simulink model "Ctrl_For_HRV_20260625_before_guidance_fix"  (R2024b)
settings: Solver=ode4  StartTime=0.0  StopTime=300  FixedStep=0.02  RelTol=1e-3
InitFcn:
  | Parameter;
values from neighbouring files (symbols this model uses):
  h_alpha = h_1    (= 0.02)    [Parameter.m]
  h_beta = h_1    (= 0.02)    [Parameter.m]
  h_miu = h_1    (= 0.02)    [Parameter.m]
  h_p = h_1    (= 0.02)    [Parameter.m]
  h_q = h_1    (= 0.02)    [Parameter.m]
  h_r = h_1    (= 0.02)    [Parameter.m]
  r_alpha = r_1    (= 0.04)    [Parameter.m]
  r_beta = r_1    (= 0.04)    [Parameter.m]
  r_miu = r_3    (= 0.03)    [Parameter.m]
  r_p = r_2    (= 1.28)    [Parameter.m]
  r_q = r_2    (= 1.28)    [Parameter.m]
  r_r = r_2    (= 1.28)    [Parameter.m]
  xishu = 0    [Parameter.m]
  xishu_D_0 = 0.3    [Parameter.m]
  xishu_L_0 = 0.2    [Parameter.m]
  xishu_l_0 = 0.23    [Parameter.m]
  xishu_m_0 = 0.17    [Parameter.m]
  xishu_n_0 = 0.09    [Parameter.m]
  xishu_Y_0 = 0.14    [Parameter.m]
undefined symbols (not defined in the file or in its folder): CCI_DUI_AngleRate_Controller, CCI_DUI_FlowAngle_Controller, fhan, PNG_2026_6_23
libraries: simulink x12
(part 2 of 2)

== matlab function Ctrl_For_HRV_20260625_before_guidance_fix/PNG/MATLAB Function1 ==
  data: ny_cmd input; alpha_cmd output; nz_cmd input; miu_cmd output; Q input; H input; Ma input; miu_last input
function [alpha_cmd, miu_cmd] = fcn(ny_cmd,nz_cmd,Q, H, Ma, miu_last)
%%%%%%%%%该函数的作用为将过载指令转化为攻角指令与倾侧角指令
%%
%参数设置
S = 334.73;
m = 63504;
earth_r = 6371000;
g0 = 9.8060;
R = earth_r+H; %R为地心距
g = (earth_r/R)^2*g0;
%% ===== 倾侧角 =====
nL=sqrt(ny_cmd^2+nz_cmd^2);
if nL <1e-4
    miu_cmd = miu_last;
else
    % atan2(y, z)，对应：
    % ny_cmd = n_lift_cmd * sin(miu_cmd)
    % nz_cmd = n_lift_cmd * cos(miu_cmd)
    miu_raw = atan2(ny_cmd, nz_cmd)

    % ===== 倾侧角连续化处理，避免 +pi/-pi 跳变 =====
    d_miu = miu_raw - miu_last;
    d_miu = mod(d_miu + pi, 2*pi) - pi;

    miu_cmd = miu_last + d_miu;
end
miu_cmd = mod(miu_cmd + pi, 2*pi) - pi;
% miu_cmd = -miu_cmd;
% miu_cmd = atan2(-ny_cmd, nz_cmd);

% if abs(miu_cmd) > pi / 2
%     miu_cmd = atan2(sin(miu_cmd - sign(miu_cmd) * pi), ...
%                 cos(miu_cmd - sign(miu_cmd) * pi));
%     % nL = -nL;
% else
%     miu_cmd = miu_cmd;
%     % nL = nL;
% end
%% ===== 攻角 =====
% C_L_alpha = (-8.19e-2)+(4.7e-2)*Ma+(1.86e-2)*alpha_deg-(4.73e-4)*(alpha_deg*Ma)-(9.19e-3)*Ma^2-(1.52e-4)*alpha_deg^2+(5.99e-7)*(alpha_deg*Ma)^2+(7.74e-4)*Ma^3+(4.08e-6)*alpha_deg^3-(2.93e-5)*Ma^4+(4.12e-7)*Ma^5;
% C_L_delta_a = (-1.45e-5)+(1.01e-4)*alpha_deg+(7.10e-6)*Ma-(4.14e-4)*delta_a-(3.51e-6)*(alpha_deg*delta_a)+(4.70e-6)*(alpha_deg*Ma)+(8.72e-6)*(Ma*delta_a)-(1.70e-7)*(alpha_deg*Ma)*delta_a;
% C_L_delta_e = (-1.45e-5)+(1.01e-4)*alpha_deg+(7.10e-6)*Ma-(4.14e-4)*delta_e-(3.51e-6)*(alpha_deg*delta_e)+(4.70e-6)*(alpha_deg*Ma)+(8.72e-6)*(Ma*delta_e)-(1.70e-7)*(alpha_deg*Ma)*delta_e;

%单位是角度
alpha_min = -30;
alpha_max = 30;

% CL_func = @(alpha_deg) (-8.19e-2)+(4.7e-2)*Ma+(1.86e-2)*alpha_deg-(4.73e-4)*(alpha_deg*Ma)-(9.19e-3)*Ma^2-(1.52e-4)*alpha_deg^2+(5.99e-7)*(alpha_deg*Ma)^2+(7.74e-4)*Ma^3+(4.08e-6)*alpha_deg^3-(2.93e-5)*Ma^4+(4.12e-7)*Ma^5 + ...
%                         (-1.45e-5)+(1.01e-4)*alpha_deg+(7.10e-6)*Ma-(4.14e-4)*delta_a-(3.51e-6)*(alpha_deg*delta_a)+(4.70e-6)*(alpha_deg*Ma)+(8.72e-6)*(Ma*delta_a)-(1.70e-7)*(alpha_deg*Ma)*delta_a + ...
%                         (-1.45e-5)+(1.01e-4)*alpha_deg+(7.10e-6)*Ma-(4.14e-4)*delta_e-(3.51e-6)*(alpha_deg*delta_e)+(4.70e-6)*(alpha_deg*Ma)+(8.72e-6)*(Ma*delta_e)-(1.70e-7)*(alpha_deg*Ma)*delta_e;

CL_func = @(alpha_deg) (-8.19e-2)+(4.7e-2)*Ma+(1.86e-2)*alpha_deg-(4.73e-4)*(alpha_deg*Ma)-(9.19e-3)*Ma^2-(1.52e-4)*alpha_deg^2+(5.99e-7)*(alpha_deg*Ma)^2+(7.74e-4)*Ma^3+(4.08e-6)*alpha_deg^3-(2.93e-5)*Ma^4+(4.12e-7)*Ma^5;
CL_min = CL_func(alpha_min);
CL_max = CL_func(alpha_max);

% ===== 目标CL =====

CL_cmd = nL*m*g/(Q*S);

% ===== 限制CL（关键）=====
CL_cmd = min(max(CL_cmd, CL_min), CL_max);

% ===== 求解 =====
alpha_cmd = fzero(@(a) CL_func(a) - CL_cmd, [alpha_min, alpha_max]);

%%

== matlab function Ctrl_For_HRV_20260625_before_guidance_fix/PNG/MATLAB Function2 ==
  data: V input; f_psi output; theta input; psi input; lat input; H input
function f_psi = earth_rotation(V,theta,psi,lat,H)

earth_r = 6371000;
w_e = 7.292116000000000e-05;
R = earth_r + H;
f_psi = V*cos(theta)*sin(psi)*tan(lat)/R ...
      + 2*w_e*(sin(lat)-cos(lat)*cos(psi)*tan(theta)) ...
      + w_e^2*R*cos(lat)*sin(lat)*sin(psi)/(V*cos(theta));

== matlab function Ctrl_For_HRV_20260625_before_guidance_fix/MATLAB Function2 ==
  data: position_t input; ny output; vt input; hgv_states input; theta_f input; kai_f input; nz output
function [ny, nz] = Prop_guidance(position_t, vt, hgv_states, theta_f, kai_f)
%--------------------------------------------------------------------------
% 两个平面的比例导引
% X-Y-Z 为北-天-东坐标系
% kai 在 x 轴右侧为正
%
% 输入：
%   xt, yt, zt   : 目标位置
%   gammat       : 目标航迹倾角
%   kait         : 目标航向角
%   Vt           : 目标速度
%   hgv_states   : [R, lon, lat, V, gamma, kai, x, y, z]
%   theta_f      : 期望终端弹道倾角
%   kai_f        : 期望终端航向角
%
% 输出：
%   ny           : 纵向过载
%   nz           : 侧向过载
%   out          : 中间变量，便于调试
%--------------------------------------------------------------------------

    %-----------------------------
    % 1. 读取状态量
    %-----------------------------
    H     = hgv_states(1);
    lon   = hgv_states(2); %#ok<NASGU>
    lat   = hgv_states(3);
    V     = hgv_states(4);
    gamma = hgv_states(5);
    kai   = hgv_states(6);
    x     = hgv_states(7);
    y     = hgv_states(8);
    z     = hgv_states(9);
    
    xt = position_t(1);
    yt = position_t(3);
    zt = position_t(2);
    %-----------------------------
    % 2. 常数与重力
    %-----------------------------
    earth_r = 6371000;
    g0 = 9.806000000000000;
    R = earth_r+H; %R_to_earth为地心距
    g = (earth_r/R)^2*g0;

    OMEGA_EARTH = 7.292116e-5;
    omega = OMEGA_EARTH;

    %-----------------------------
    % 3. 相对位置
    %-----------------------------
    rx = xt - x;
    ry = yt - y;
    rz = zt - z;

    %-----------------------------
    % 4. 目标速度分量
    % 这里保持你的 Python 代码逻辑，虽然后面没有直接用到
    %-----------------------------
    % vxt = Vt * cos(gammat) * cos(kait); %#ok<NASGU>
    % vyt = Vt * sin(gammat);             %#ok<NASGU>
    % vzt = Vt * cos(gammat) * sin(kait); %#ok<NASGU>
    vxt = vt(1);
    vyt = vt(3);
    vzt = vt(2);

    %-----------------------------
    % 5. 飞行器速度分量
    % 这里保持你的 Python 代码逻辑，虽然后面没有直接用到
    %-----------------------------
    vx = V * cos(gamma) * cos(kai); %#ok<NASGU>
    vy = V * sin(gamma);            %#ok<NASGU>
    vz = V * cos(gamma) * sin(kai); %#ok<NASGU>

    %-----------------------------
    % 6. 距离与视线角
    %-----------------------------
    rd = sqrt(rx^2 + ry^2 + rz^2);
    rc = sqrt(rx^2 + rz^2);

    qz = atan2(rz, rx);

    % Python 里是 atan(ry / rc)
    % MATLAB 里建议写成 atan2(ry, rc)，数值上更稳
    qy = atan2(ry, rc);

    % 如果想和 Python 完全一致，也可以改成：
    % qy = atan(ry / rc);

    %-----------------------------
    % 7. 视线角速度与距离变化率
    %-----------------------------
    qy_dot = -V * ( ...
        sin(gamma) * cos(qy) ...
        - cos(gamma) * sin(qy) * cos(kai - qz) ...
        ) / rd;

    qz_dot = -V * cos(gamma) * sin(kai - qz) / ...
        (rd * cos(qy));

    rd_dot = -V * ( ...
        cos(gamma) * cos(qy) * cos(kai - qz) ...
        + sin(gamma) * sin(qy) ...
        );

    %-----------------------------
    % 8. 剩余飞行时间估计
    %-----------------------------
    tgo = rd / abs(rd_dot);

    %-----------------------------
    % 9. 制导参数
    %-----------------------------
    k1  = 4;
    k2  = 4;
    k11 = 2.5;
    k21 = 5; %#ok<NASGU>

    %-----------------------------
    % 10. 航迹倾角与航向角指令变化率
    %-----------------------------
    gamma_dot = k1 * qy_dot * cos(qz - kai);

    % gamma_dot = k1 * qy_dot * cos(qz - kai) ...
    % - k11 * (theta_f - qy) / tgo;
    kai_dot = k2 * qz_dot ...
        - k2 * qy_dot * tan(gamma) * sin(qz - kai);

    % 你 Python 代码里这一项被注释掉了：
    % kai_dot = kai_dot + k21 * (kai_f - kai) / tgo;

    %-----------------------------
    % 11. 地球自转修正项
    %-----------------------------
    epi_gamma = 2 * omega * cos(lat) * sin(kai) ...
        + omega^2 * R * ( ...
        cos(lat)^2 * cos(gamma) ...
        + cos(lat) * sin(lat) * cos(kai) * sin(gamma) ...
        ) / V;

    epi_kai = 2 * omega * ( ...
        sin(lat) ...
        - cos(lat) * cos(kai) * tan(gamma) ...
        ) ...
        + omega^2 * R * cos(lat) * sin(lat) * sin(kai) / ...
        (V * cos(gamma));

    %-----------------------------
    % 12. 纵向与侧向过载
    %-----------------------------
    ny = ( ...
        gamma_dot ...
        + g * cos(gamma) / V ...
        - V * cos(gamma) / R ...
        - epi_gamma ...
        ) * V / g;

    nz = ( ...
        kai_dot ...
        - V * cos(gamma) * tan(lat) * sin(kai) / R ...
        - epi_kai ...
        ) * V * cos(gamma) / g;

    % %-----------------------------
    % % 13. 输出中间变量，便于检查
    % %-----------------------------
    % out = struct();
    % 
    % out.rx = rx;
    % out.ry = ry;
    % out.rz = rz;
    % 
    % out.rd = rd;
    % out.rc = rc;
    % 
    % out.qy = qy;
    % out.qz = qz;
    % 
    % out.qy_dot = qy_dot;
    % out.qz_dot = qz_dot;
    % out.rd_dot = rd_dot;
    % out.tgo = tgo;
    % 
    % out.gamma_dot = gamma_dot;
    % out.kai_dot = kai_dot;
    % 
    % out.epi_gamma = epi_gamma;
    % out.epi_kai = epi_kai;
    % 
    % out.ny = ny;
    % out.nz = nz;

end
